simulink model "open_differential"  (R2024b)
settings: Solver=FixedStepDiscrete  StartTime=0.0  StopTime=10.0  RelTol=1e-3
libraries: slpidlib x2, simulink x2
settings Model: Creator=chris  LastModifiedBy=chris
settings OptimizationCC: DefaultParameterBehavior=Inlined  UseDivisionForNetSlopeComputation=on  GainParamInheritBuiltInType=on  UseFloatMulNetSlope=on  InlineInvariantSignals=on  PassReuseOutputArgsAs=Individual arguments  ZeroExternalMemoryAtStartup=off  ZeroInternalMemoryAtStartup=off  NoFixptDivByZeroProtection=on  EfficientFloat2IntCast=on  LifeSpan=1  OptimizeBlockOrder=speed  DifferentSizesBufferReuse=on  EfficientTunableParamExpr=on
settings DebuggingCC: ParameterTunabilityLossMsg=error
settings HardwareCC: ProdBitPerPointer=32  ProdBitPerSizeT=32  ProdBitPerPtrDiffT=32  ProdLargestAtomicInteger=Long  ProdLargestAtomicFloat=Double  ProdWordSize=32  ProdLongLongMode=on  ProdHWDeviceType=ARM Compatible->ARM Cortex-M
settings SFSimCC: MATLABDynamicMemAlloc=off
settings RTWCC: Description=Embedded Coder  SystemTargetFile=ert.tlc  TemplateMakefile=ert_default_tmf
settings CodeAppCC: ForceParamTrailComments=on  IgnoreCustomStorageClasses=off  OperatorAnnotations=on  SimulinkDataObjDesc=on  SFDataObjDesc=on  CustomSymbolStrGlobalVar=rt$N$M  CustomSymbolStrType=$N$M  CustomSymbolStrFcn=$N$M$F  CustomSymbolStrMacro=$N$M  InsertBlockDesc=on
settings ERTTargetCC: TargetLangStandard=C99 (ISO)  GenerateSampleERTMain=on  IncludeMdlTerminateFcn=off  CombineSignalStateStructs=on  SupportAbsoluteTime=off  SupportComplex=off  SupportNonInlinedSFcns=on  ERTCustomFileTemplate=example_file_process.tlc  ERTFilePackagingFormat=CompactWithDataFile

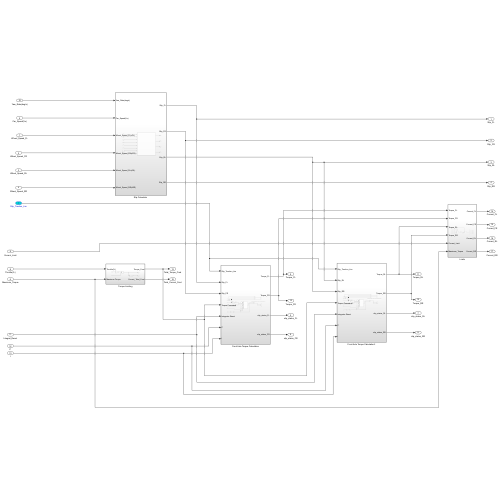
[thumbnail: Simulink's stored preview of the top-level diagram]
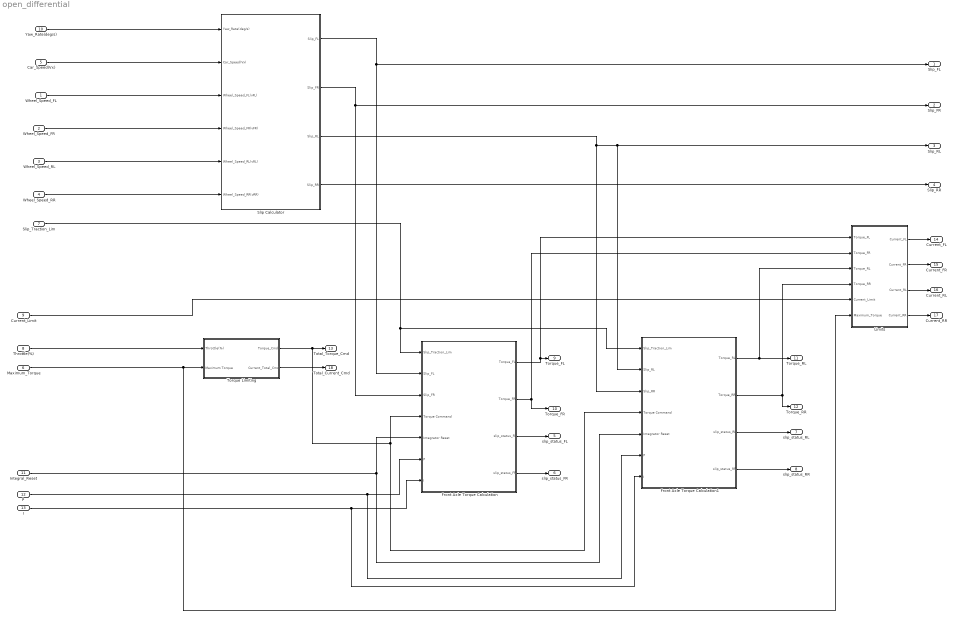
== system open_differential ==
  Wheel_Speed_FL : Inport
  Wheel_Speed_FR : Inport  Port=2
  Wheel_Speed_RL : Inport  Port=3
  Wheel_Speed_RR : Inport  Port=4
  Car_Speed(Vx) : Inport  Port=5
  Maximum_Torque : Inport  Port=6
  Slip_Traction_Lim : Inport  Port=7
  Throttle(%) : Inport  Port=8
  Current_Limit : Inport  Port=9
  Yaw_Rate(deg/s) : Inport  Port=10
  Integral_Reset : Inport  Port=11
  P : Inport  Port=12
  I : Inport  Port=13
  Front Axle Torque Calculation : Subsystem
  Front Axle Torque Calculation1 : Subsystem
  Limits : Subsystem
  "Slip Calculator " : Subsystem
  Torque Limiting : Subsystem
  Slip_FL : Outport
  Slip_FR : Outport  Port=2
  Slip_RL : Outport  Port=3
  Slip_RR : Outport  Port=4
  slip_status_FL : Outport  Port=5
  slip_status_FR : Outport  Port=6
  slip_status_RL : Outport  Port=7
  slip_status_RR : Outport  Port=8
  Torque_FL : Outport  Port=9
  Torque_FR : Outport  Port=10
  Torque_RL : Outport  Port=11
  Torque_RR : Outport  Port=12
  Total_Torque_Cmd : Outport  Port=13
  Current_FL : Outport  Port=14
  Current_FR : Outport  Port=15
  Current_RL : Outport  Port=16
  Current_RR : Outport  Port=17
  Total_Current_Cmd : Outport  Port=18
  wires:
  Yaw_Rate(deg/s)/1 -> "Slip Calculator "/1(Yaw_Rate(deg/s))
  Front Axle Torque Calculation1/1(Torque_RL) -> Torque_RL/1, Limits/3(Torque_RL)
  Front Axle Torque Calculation1/2(Torque_RR) -> Torque_RR/1, Limits/4(Torque_RR)
  Front Axle Torque Calculation1/4(slip_status_RR) -> slip_status_RR/1
  Torque Limiting/2(Current_Total_Cmd) -> Total_Current_Cmd/1
  "Slip Calculator "/3(Slip_RL) -> Front Axle Torque Calculation1/3(Slip_RR), Front Axle Torque Calculation1/2(Slip_RL), Slip_RL/1
  Slip_Traction_Lim/1 -> Front Axle Torque Calculation1/1(Slip_Traction_Lim), Front Axle Torque Calculation/1(Slip_Traction_Lim)
  Torque Limiting/1(Torque_Cmd) -> Front Axle Torque Calculation1/4(Torque Command), Front Axle Torque Calculation/4(Torque Command), Total_Torque_Cmd/1
  "Slip Calculator "/2(Slip_FR) -> Front Axle Torque Calculation/3(Slip_FR), Slip_FR/1
  Wheel_Speed_FL/1 -> "Slip Calculator "/3(Wheel_Speed_FL(vFL))
  Front Axle Torque Calculation/2(Torque_FR) -> Limits/2(Torque_FR), Torque_FR/1
  Front Axle Torque Calculation1/3(slip_status_RL) -> slip_status_RL/1
  "Slip Calculator "/4(Slip_RR) -> Slip_RR/1
  Wheel_Speed_RR/1 -> "Slip Calculator "/6(Wheel_Speed_RR(vRR))
  Wheel_Speed_RL/1 -> "Slip Calculator "/5(Wheel_Speed_RL(vRL))
  Car_Speed(Vx)/1 -> "Slip Calculator "/2(Car_Speed(Vx))
  Limits/1(Current_FL) -> Current_FL/1
  Limits/3(Current_RL) -> Current_RL/1
  Limits/4(Current_RR) -> Current_RR/1
  Maximum_Torque/1 -> Torque Limiting/2(Maximum Torque), Limits/6(Maximum_Torque)
  Current_Limit/1 -> Limits/5(Current_Limit)
  "Slip Calculator "/1(Slip_FL) -> Front Axle Torque Calculation/2(Slip_FL), Slip_FL/1
  Front Axle Torque Calculation/3(slip_status_FL) -> slip_status_FL/1
  Throttle(%)/1 -> Torque Limiting/1(Throttle(%))
  Front Axle Torque Calculation/1(Torque_FL) -> Limits/1(Torque_FL), Torque_FL/1
  Wheel_Speed_FR/1 -> "Slip Calculator "/4(Wheel_Speed_FR(vFR))
  Front Axle Torque Calculation/4(slip_status_FR) -> slip_status_FR/1
  Limits/2(Current_FR) -> Current_FR/1
  Integral_Reset/1 -> Front Axle Torque Calculation1/5(Integrator Reset), Front Axle Torque Calculation/5(Integrator Reset)
  P/1 -> Front Axle Torque Calculation/6(P), Front Axle Torque Calculation1/6(P)
  I/1 -> Front Axle Torque Calculation/7(I), Front Axle Torque Calculation1/7(I)

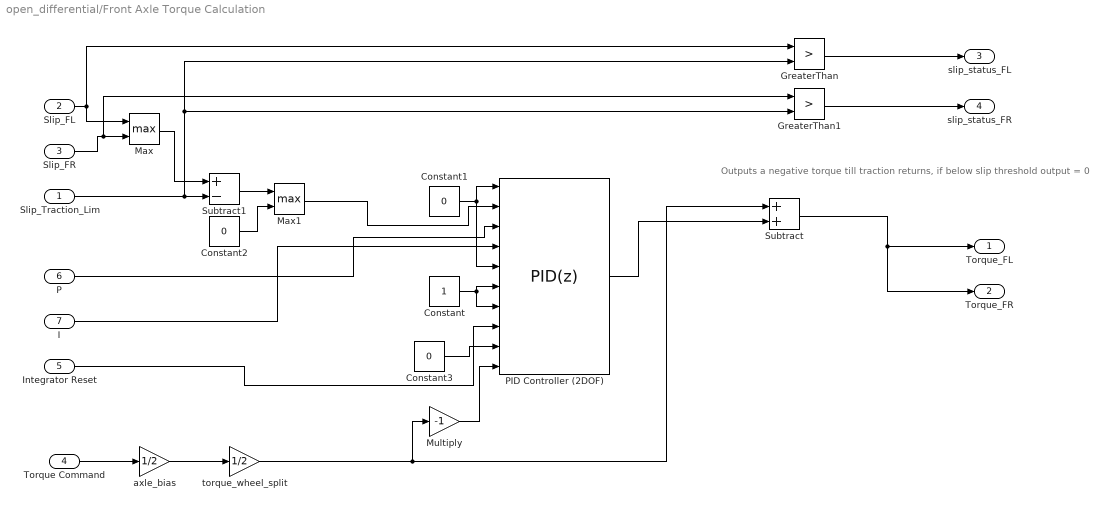
== system open_differential/Front Axle Torque Calculation ==
  note: Outputs a negative torque till traction returns, if below slip threshold output = 0
  Slip_Traction_Lim : Inport
  Slip_FL : Inport  Port=2
  Slip_FR : Inport  Port=3
  Torque Command : Inport  Port=4
  Integrator Reset : Inport  Port=5
  P : Inport  Port=6
  I : Inport  Port=7
  Constant : Constant
  Constant1 : Constant  Value=0
  Constant2 : Constant  Value=0
  Constant3 : Constant  Value=0
  GreaterThan : RelationalOperator  Operator=>  OutDataTypeStr=boolean  RndMeth=Simplest  InputSameDT=off
  GreaterThan1 : RelationalOperator  Operator=>  OutDataTypeStr=boolean  RndMeth=Simplest  InputSameDT=off
  Max : MinMax  Function=max  Inputs=2
  Max1 : MinMax  Function=max  Inputs=2
  Multiply : Gain  Gain=-1
  PID Controller (2DOF) : slpidlib/PID Controller (2DOF)  Controller=PID  Form=Parallel  TimeDomain=Discrete-time  UseExternalTs=off  SampleTime=0.010  IntegratorMethod=Forward Euler  FilterMethod=Forward Euler  ControllerParametersSource=external  P=5  I=0.5  UseKiTs=off  D=0  UseExternalDerivativeSource=off  N=100  UseFilter=off  b=1  c=1  TunerSelectOption=Transfer Function Based (PID Tuner App)  ZeroCross=off  InitialConditionSource=internal  InitialConditionForIntegrator=0  InitialConditionForFilter=0  DifferentiatorICPrevScaledInput=0  ExternalReset=rising  TrackingMode=off  Kt=1  LimitOutput=on  SatLimitsSource=external  UpperSaturationLimit=30.84  LowerSaturationLimit=0  LinearizeAsGain=off  AntiWindupMode=clamping  Kb=1  LimitIntegrator=off  UpperIntegratorSaturationLimit=inf  LowerIntegratorSaturationLimit=-inf  POutMin=[]  POutMax=[]  IOutMin=[]  IOutMax=[]  DOutMin=[]  DOutMax=[]  NOutMin=[]  NOutMax=[]  bOutMin=[]  bOutMax=[]  cOutMin=[]  cOutMax=[]  SumOutMin=[]  SumOutMax=[]  SaturationOutMin=[]  SaturationOutMax=[]  PParamMin=[]  PParamMax=[]  IParamMin=[]  IParamMax=[]  DParamMin=[]  DParamMax=[]  NParamMin=[]  NParamMax=[]  bParamMin=[]  bParamMax=[]  cParamMin=[]  cParamMax=[]  KbParamMin=[]  KbParamMax=[]  KtParamMin=[]  KtParamMax=[]  KbOutMin=[]  KbOutMax=[]  KtOutMin=[]  KtOutMax=[]  IntegratorOutMin=[]  IntegratorOutMax=[]  FilterOutMin=[]  FilterOutMax=[]  SumI1OutMin=[]  SumI1OutMax=[]  SumI2OutMin=[]  SumI2OutMax=[]  SumI3OutMin=[]  SumI3OutMax=[]  SumI4OutMin=[]  SumI4OutMax=[]  SumDOutMin=[]  SumDOutMax=[]  Sum1OutMin=[]  Sum1OutMax=[]  Sum2OutMin=[]  Sum2OutMax=[]  Sum3OutMin=[]  Sum3OutMax=[]  DifferentiatorOutMin=[]  DifferentiatorOutMax=[]  FilterDiffOutCoefMin=[]  FilterDiffOutCoefMax=[]  ReciprocalOutMin=[]  ReciprocalOutMax=[]  SumDenOutMin=[]  SumDenOutMax=[]  SumNumOutMin=[]  SumNumOutMax=[]  DivideOutMin=[]  DivideOutMax=[]  UdiffTsProdOutMin=[]  UdiffTsProdOutMax=[]  NTsProdOutMin=[]  NTsProdOutMax=[]  UintegralTsProdOutMin=[]  UintegralTsProdOutMax=[]  UngainTsProdOutMin=[]  UngainTsProdOutMax=[]  ClampingZeroOutDataTypeStr=Inherit: Inherit via back propagation  ClampingZeroOutMin=[]  ClampingZeroOutMax=[]  FilterDenConstantOutDataTypeStr=Inherit: Inherit via back propagation  FilterDenConstantOutMin=[]  FilterDenConstantOutMax=[]  PCopyOutDataTypeStr=Inherit: Inherit via back propagation  PCopyOutMin=[]  PCopyOutMax=[]  NCopyOutDataTypeStr=Inherit: Inherit via back propagation  NCopyOutMin=[]  NCopyOutMax=[]  IntegratorContinuousStateAttributes=''  IntegratorStateMustResolveToSignalObject=off  IntegratorRTWStateStorageClass=Auto  FilterContinuousStateAttributes=''  FilterStateMustResolveToSignalObject=off  FilterRTWStateStorageClass=Auto  ParallelPVariant=ExternalParameters  IdealPVariant=Disabled  IVariant=ExternalParameters  DVariant=ExternalParameters  bVariant=ExternalParameters  cVariant=ExternalParameters  IntegratorVariant=Discrete  SatVariant=External  AWVariant=DiscClampingParallel  PCopyVariant=Disabled  TRVariant=Disabled  FdbkBlocksVariant=Forward  IdealPFdbkVariant=Disabled  SatFdbkVariant=Disabled  DerivativeFilterVariant=Differentiator  NVariant=Passthrough  NCopyVariant=Disabled_SignalSpec  FilterICVariant=InternalICsDifferentiator  IntegratorICVariant=InternalICs  ExternalResetVariant=ExternalReset  TRSumVariant=Passthrough  SumFdbkVariant=Disabled  SumVariant=Sum_PID  TsampFilterVariant=InternalTs  TsampNgainVariant=Passthrough  TsampIntegralVariant=Disabled_SignalSpec  ExternalSaturationOutDataTypeStr=Inherit: Same as second input  DerivativeSourceVariant=ErrorSignal  PreIntVariant=InternalPreInt
  Subtract : Sum
  Subtract1 : Sum  Inputs=+-
  axle_bias : Gain  Gain=1/2
  torque_wheel_split : Gain  Gain=1/2
  Torque_FL : Outport
  Torque_FR : Outport  Port=2
  slip_status_FL : Outport  Port=3
  slip_status_FR : Outport  Port=4
  wires:
  Torque Command/1 -> axle_bias/1
  axle_bias/1 -> torque_wheel_split/1
  Integrator Reset/1 -> PID Controller (2DOF)/8
  torque_wheel_split/1 -> Multiply/1, Subtract/1
  PID Controller (2DOF)/1 -> Subtract/2
  Subtract/1 -> Torque_FR/1, Torque_FL/1
  Slip_FR/1 -> GreaterThan1/1, Max/2
  Slip_FL/1 -> GreaterThan/1, Max/1
  Constant1/1 -> PID Controller (2DOF)/5, PID Controller (2DOF)/1
  Subtract1/1 -> Max1/1
  Max1/1 -> PID Controller (2DOF)/2
  Constant2/1 -> Max1/2
  Slip_Traction_Lim/1 -> GreaterThan/2, GreaterThan1/2, Subtract1/2
  Max/1 -> Subtract1/1
  Constant3/1 -> PID Controller (2DOF)/9
  Multiply/1 -> PID Controller (2DOF)/10
  GreaterThan/1 -> slip_status_FL/1
  GreaterThan1/1 -> slip_status_FR/1
  P/1 -> PID Controller (2DOF)/3
  I/1 -> PID Controller (2DOF)/4
  Constant/1 -> PID Controller (2DOF)/7, PID Controller (2DOF)/6

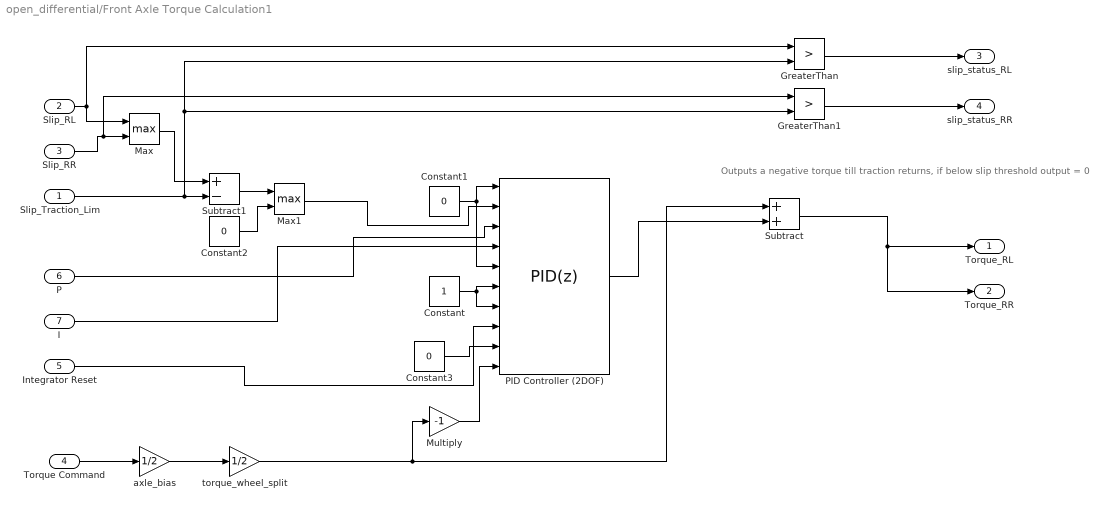
== system open_differential/Front Axle Torque Calculation1 ==
  note: Outputs a negative torque till traction returns, if below slip threshold output = 0
  Slip_Traction_Lim : Inport
  Slip_RL : Inport  Port=2
  Slip_RR : Inport  Port=3
  Torque Command : Inport  Port=4
  Integrator Reset : Inport  Port=5
  P : Inport  Port=6
  I : Inport  Port=7
  Constant : Constant
  Constant1 : Constant  Value=0
  Constant2 : Constant  Value=0
  Constant3 : Constant  Value=0
  GreaterThan : RelationalOperator  Operator=>  OutDataTypeStr=boolean  RndMeth=Simplest  InputSameDT=off
  GreaterThan1 : RelationalOperator  Operator=>  OutDataTypeStr=boolean  RndMeth=Simplest  InputSameDT=off
  Max : MinMax  Function=max  Inputs=2
  Max1 : MinMax  Function=max  Inputs=2
  Multiply : Gain  Gain=-1
  PID Controller (2DOF) : slpidlib/PID Controller (2DOF)  Controller=PID  Form=Parallel  TimeDomain=Discrete-time  UseExternalTs=off  SampleTime=0.010  IntegratorMethod=Forward Euler  FilterMethod=Forward Euler  ControllerParametersSource=external  P=5  I=0.5  UseKiTs=off  D=0  UseExternalDerivativeSource=off  N=100  UseFilter=off  b=1  c=1  TunerSelectOption=Transfer Function Based (PID Tuner App)  ZeroCross=off  InitialConditionSource=internal  InitialConditionForIntegrator=0  InitialConditionForFilter=0  DifferentiatorICPrevScaledInput=0  ExternalReset=rising  TrackingMode=off  Kt=1  LimitOutput=on  SatLimitsSource=external  UpperSaturationLimit=30.84  LowerSaturationLimit=0  LinearizeAsGain=off  AntiWindupMode=clamping  Kb=1  LimitIntegrator=off  UpperIntegratorSaturationLimit=inf  LowerIntegratorSaturationLimit=-inf  POutMin=[]  POutMax=[]  IOutMin=[]  IOutMax=[]  DOutMin=[]  DOutMax=[]  NOutMin=[]  NOutMax=[]  bOutMin=[]  bOutMax=[]  cOutMin=[]  cOutMax=[]  SumOutMin=[]  SumOutMax=[]  SaturationOutMin=[]  SaturationOutMax=[]  PParamMin=[]  PParamMax=[]  IParamMin=[]  IParamMax=[]  DParamMin=[]  DParamMax=[]  NParamMin=[]  NParamMax=[]  bParamMin=[]  bParamMax=[]  cParamMin=[]  cParamMax=[]  KbParamMin=[]  KbParamMax=[]  KtParamMin=[]  KtParamMax=[]  KbOutMin=[]  KbOutMax=[]  KtOutMin=[]  KtOutMax=[]  IntegratorOutMin=[]  IntegratorOutMax=[]  FilterOutMin=[]  FilterOutMax=[]  SumI1OutMin=[]  SumI1OutMax=[]  SumI2OutMin=[]  SumI2OutMax=[]  SumI3OutMin=[]  SumI3OutMax=[]  SumI4OutMin=[]  SumI4OutMax=[]  SumDOutMin=[]  SumDOutMax=[]  Sum1OutMin=[]  Sum1OutMax=[]  Sum2OutMin=[]  Sum2OutMax=[]  Sum3OutMin=[]  Sum3OutMax=[]  DifferentiatorOutMin=[]  DifferentiatorOutMax=[]  FilterDiffOutCoefMin=[]  FilterDiffOutCoefMax=[]  ReciprocalOutMin=[]  ReciprocalOutMax=[]  SumDenOutMin=[]  SumDenOutMax=[]  SumNumOutMin=[]  SumNumOutMax=[]  DivideOutMin=[]  DivideOutMax=[]  UdiffTsProdOutMin=[]  UdiffTsProdOutMax=[]  NTsProdOutMin=[]  NTsProdOutMax=[]  UintegralTsProdOutMin=[]  UintegralTsProdOutMax=[]  UngainTsProdOutMin=[]  UngainTsProdOutMax=[]  ClampingZeroOutDataTypeStr=Inherit: Inherit via back propagation  ClampingZeroOutMin=[]  ClampingZeroOutMax=[]  FilterDenConstantOutDataTypeStr=Inherit: Inherit via back propagation  FilterDenConstantOutMin=[]  FilterDenConstantOutMax=[]  PCopyOutDataTypeStr=Inherit: Inherit via back propagation  PCopyOutMin=[]  PCopyOutMax=[]  NCopyOutDataTypeStr=Inherit: Inherit via back propagation  NCopyOutMin=[]  NCopyOutMax=[]  IntegratorContinuousStateAttributes=''  IntegratorStateMustResolveToSignalObject=off  IntegratorRTWStateStorageClass=Auto  FilterContinuousStateAttributes=''  FilterStateMustResolveToSignalObject=off  FilterRTWStateStorageClass=Auto  ParallelPVariant=ExternalParameters  IdealPVariant=Disabled  IVariant=ExternalParameters  DVariant=ExternalParameters  bVariant=ExternalParameters  cVariant=ExternalParameters  IntegratorVariant=Discrete  SatVariant=External  AWVariant=DiscClampingParallel  PCopyVariant=Disabled  TRVariant=Disabled  FdbkBlocksVariant=Forward  IdealPFdbkVariant=Disabled  SatFdbkVariant=Disabled  DerivativeFilterVariant=Differentiator  NVariant=Passthrough  NCopyVariant=Disabled_SignalSpec  FilterICVariant=InternalICsDifferentiator  IntegratorICVariant=InternalICs  ExternalResetVariant=ExternalReset  TRSumVariant=Passthrough  SumFdbkVariant=Disabled  SumVariant=Sum_PID  TsampFilterVariant=InternalTs  TsampNgainVariant=Passthrough  TsampIntegralVariant=Disabled_SignalSpec  ExternalSaturationOutDataTypeStr=Inherit: Same as second input  DerivativeSourceVariant=ErrorSignal  PreIntVariant=InternalPreInt
  Subtract : Sum
  Subtract1 : Sum  Inputs=+-
  axle_bias : Gain  Gain=1/2
  torque_wheel_split : Gain  Gain=1/2
  Torque_RL : Outport
  Torque_RR : Outport  Port=2
  slip_status_RL : Outport  Port=3
  slip_status_RR : Outport  Port=4
  wires:
  Torque Command/1 -> axle_bias/1
  axle_bias/1 -> torque_wheel_split/1
  Integrator Reset/1 -> PID Controller (2DOF)/8
  torque_wheel_split/1 -> Multiply/1, Subtract/1
  PID Controller (2DOF)/1 -> Subtract/2
  Subtract/1 -> Torque_RR/1, Torque_RL/1
  Slip_RR/1 -> GreaterThan1/1, Max/2
  Slip_RL/1 -> GreaterThan/1, Max/1
  Constant1/1 -> PID Controller (2DOF)/5, PID Controller (2DOF)/1
  Subtract1/1 -> Max1/1
  Max1/1 -> PID Controller (2DOF)/2
  Constant2/1 -> Max1/2
  Slip_Traction_Lim/1 -> GreaterThan/2, GreaterThan1/2, Subtract1/2
  Max/1 -> Subtract1/1
  Constant3/1 -> PID Controller (2DOF)/9
  Multiply/1 -> PID Controller (2DOF)/10
  GreaterThan/1 -> slip_status_RL/1
  GreaterThan1/1 -> slip_status_RR/1
  P/1 -> PID Controller (2DOF)/3
  I/1 -> PID Controller (2DOF)/4
  Constant/1 -> PID Controller (2DOF)/7, PID Controller (2DOF)/6

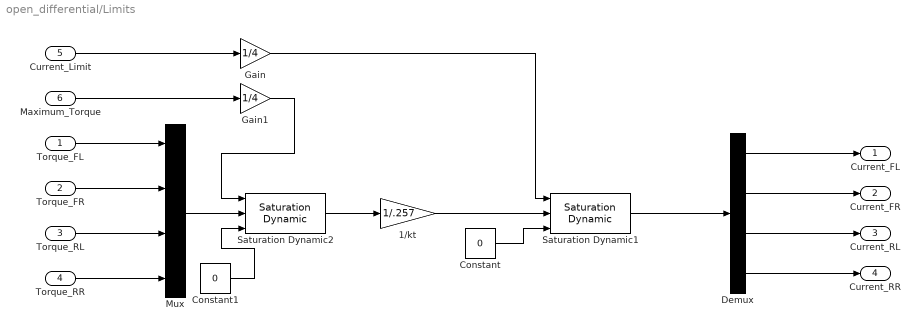
== system open_differential/Limits ==
  Torque_FL : Inport
  Torque_FR : Inport  Port=2
  Torque_RL : Inport  Port=3
  Torque_RR : Inport  Port=4
  Current_Limit : Inport  Port=5
  Maximum_Torque : Inport  Port=6
  1/kt : Gain  Gain=1/.257
  Constant : Constant  Value=0
  Constant1 : Constant  Value=0
  Demux : Demux
  Gain : Gain  Gain=1/4
  Gain1 : Gain  Gain=1/4
  Mux : Mux
  Saturation Dynamic1 : simulink/Discontinuities/Saturation Dynamic  OutMin=[]  OutMax=[]  OutDataTypeStr=Inherit: Same as second input  OutDataType=fixdt(1, 16)  OutScaling=2^-10  DoSatur=off
  Saturation Dynamic2 : simulink/Discontinuities/Saturation Dynamic  OutMin=[]  OutMax=[]  OutDataTypeStr=Inherit: Same as second input  OutDataType=fixdt(1, 16)  OutScaling=2^-10  DoSatur=off
  Current_FL : Outport
  Current_FR : Outport  Port=2
  Current_RL : Outport  Port=3
  Current_RR : Outport  Port=4
  wires:
  Torque_FR/1 -> Mux/2
  Torque_FL/1 -> Mux/1
  Torque_RL/1 -> Mux/3
  Torque_RR/1 -> Mux/4
  Constant/1 -> Saturation Dynamic1/3
  Demux/1 -> Current_FL/1
  Demux/2 -> Current_FR/1
  Demux/3 -> Current_RL/1
  Demux/4 -> Current_RR/1
  1/kt/1 -> Saturation Dynamic1/2
  Saturation Dynamic1/1 -> Demux/1
  Current_Limit/1 -> Gain/1
  Gain/1 -> Saturation Dynamic1/1
  Maximum_Torque/1 -> Gain1/1
  Mux/1 -> Saturation Dynamic2/2
  Saturation Dynamic2/1 -> 1/kt/1
  Gain1/1 -> Saturation Dynamic2/1
  Constant1/1 -> Saturation Dynamic2/3

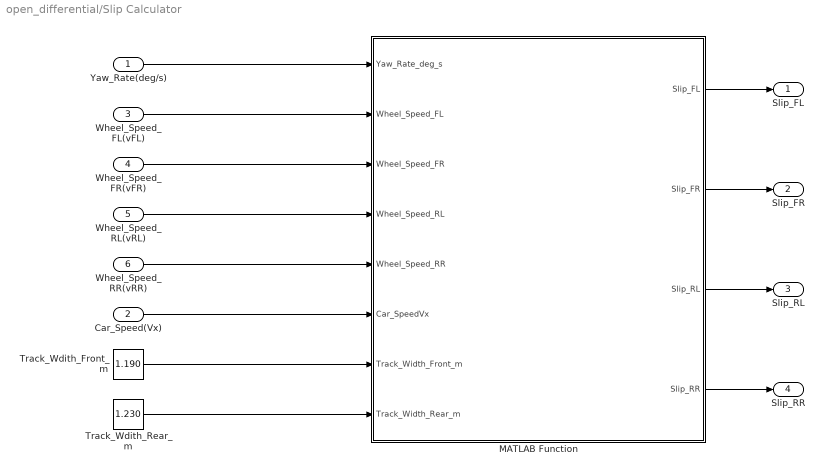
== system open_differential/Slip Calculator  ==
  Yaw_Rate(deg/s) : Inport
  Car_Speed(Vx) : Inport  Port=2
  Wheel_Speed_FL(vFL) : Inport  Port=3
  Wheel_Speed_FR(vFR) : Inport  Port=4
  Wheel_Speed_RL(vRL) : Inport  Port=5
  Wheel_Speed_RR(vRR) : Inport  Port=6
  MATLAB Function : MATLAB Function  TreatAsAtomicUnit=on
  Track_Wdith_Front_m : Constant  Value=1.190
  Track_Wdith_Rear_m : Constant  Value=1.230
  Slip_FL : Outport
  Slip_FR : Outport  Port=2
  Slip_RL : Outport  Port=3
  Slip_RR : Outport  Port=4
  wires:
  Wheel_Speed_FL(vFL)/1 -> MATLAB Function/2(Wheel_Speed_FL)
  Wheel_Speed_FR(vFR)/1 -> MATLAB Function/3(Wheel_Speed_FR)
  Wheel_Speed_RL(vRL)/1 -> MATLAB Function/4(Wheel_Speed_RL)
  Wheel_Speed_RR(vRR)/1 -> MATLAB Function/5(Wheel_Speed_RR)
  Yaw_Rate(deg/s)/1 -> MATLAB Function/1(Yaw_Rate_deg_s)
  Car_Speed(Vx)/1 -> MATLAB Function/6(Car_SpeedVx)
  Track_Wdith_Front_m/1 -> MATLAB Function/7(Track_Width_Front_m)
  Track_Wdith_Rear_m/1 -> MATLAB Function/8(Track_Width_Rear_m)
  MATLAB Function/1(Slip_FL) -> Slip_FL/1
  MATLAB Function/2(Slip_FR) -> Slip_FR/1
  MATLAB Function/3(Slip_RL) -> Slip_RL/1
  MATLAB Function/4(Slip_RR) -> Slip_RR/1

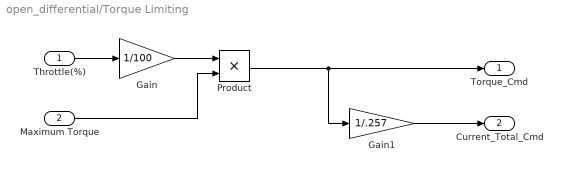
== system open_differential/Torque Limiting ==
  Throttle(%) : Inport
  Maximum Torque : Inport  Port=2
  Gain : Gain  Gain=1/100
  Gain1 : Gain  Gain=1/.257
  Product : Product
  Torque_Cmd : Outport
  Current_Total_Cmd : Outport  Port=2
  wires:
  Throttle(%)/1 -> Gain/1
  Maximum Torque/1 -> Product/2
  Gain/1 -> Product/1
  Product/1 -> Gain1/1, Torque_Cmd/1
  Gain1/1 -> Current_Total_Cmd/1

== matlab function open_differential/Slip Calculator /MATLAB Function ==
  data: Yaw_Rate_deg_s input; Slip_FL output; Wheel_Speed_FL input; Wheel_Speed_FR input; Wheel_Speed_RL input; Wheel_Speed_RR input; Car_SpeedVx input; Track_Width_Front_m input; Track_Width_Rear_m input; Slip_FR output; Slip_RL output; Slip_RR output
function [Slip_FL, Slip_FR, Slip_RL, Slip_RR] = fcn(Yaw_Rate_deg_s, Wheel_Speed_FL, Wheel_Speed_FR, Wheel_Speed_RL, Wheel_Speed_RR, Car_SpeedVx, Track_Width_Front_m, Track_Width_Rear_m)

yaw_rate_rad_s = Yaw_Rate_deg_s * (pi / 180.0);

vx_min = 0.2;

Vx = max(Car_SpeedVx, vx_min);

Vx_FL = Vx - (yaw_rate_rad_s * Track_Width_Front_m / 2.0);
Vx_FR = Vx + (yaw_rate_rad_s * Track_Width_Front_m / 2.0);
Vx_RL = Vx - (yaw_rate_rad_s * Track_Width_Rear_m / 2.0);
Vx_RR = Vx + (yaw_rate_rad_s * Track_Width_Rear_m / 2.0);

Vx_FL = max(Vx_FL, vx_min);
Vx_FR = max(Vx_FR, vx_min);
Vx_RL = max(Vx_RL, vx_min);
Vx_RR = max(Vx_RR, vx_min);

Slip_FL = max((Wheel_Speed_FL - Vx_FL) / Vx_FL, 0.0);
Slip_FR = max((Wheel_Speed_FR - Vx_FR) / Vx_FR, 0.0);
Slip_RL = max((Wheel_Speed_RL - Vx_RL) / Vx_RL, 0.0);
Slip_RR = max((Wheel_Speed_RR - Vx_RR) / Vx_RR, 0.0);

end
